simulink model "TxSteering_RxMVDR_4x4_HDL_IQ"  (R2020a)
settings: Solver=FixedStepDiscrete  StartTime=0.0  StopTime=stoptime*0 + inf  RelTol=1e-3
PreLoadFcn:
  | load('iq_bus_obj.mat');
  | model_init
InitFcn:
  | model_init
model workspace (MAT data in the model file):
  socvcb : containers.Map (value not decoded)
values from neighbouring files (symbols this model uses):
  BackSubstitutePrototype = fi(0, matrixdivbacksub_dt)    [model_init.m]
  DataSampleRate = ConverterSampleRate/DecimInterpFactor    (= 245760000)    [model_init.m]
  fc = ConverterSampleRate/4    (= 491520000)    [model_init.m]
  FPGAClkRate = DataSampleRate/VectorSamplingFactor    (= 245760000)    [model_init.m]
  matrixDivDelay = NumberOfCORDICIterations*10 + 86    [model_init.m]
  movavg_bitshift = nextpow2(sqrt(windowSize))    [model_init.m]
  mvdrPipelineDelay = covMatDelay+movAvgDelay+matrixDivDelay+normResponseDelay    [model_init.m]
  NCO_bits = 14    [model_init.m]
  numArrayElements = 4    [model_init.m]
  NumberOfCORDICIterations = matrixdivin_dt.WordLength - 1    [model_init.m]
  S2MM_frame_size = FrameSize*4    (= 40000)    [host_io_init.m]    (also in model_init.m = 1000)
  windowSize = 1024    [model_init.m]
undefined symbols (not defined in the file or in its folder): Fo, Fs, N, physconst
libraries: hdlsllib x268, simulink x53, dspsolvers x1, embreciprocals x1, dsphdlsigops x1
(part 3 of 12)

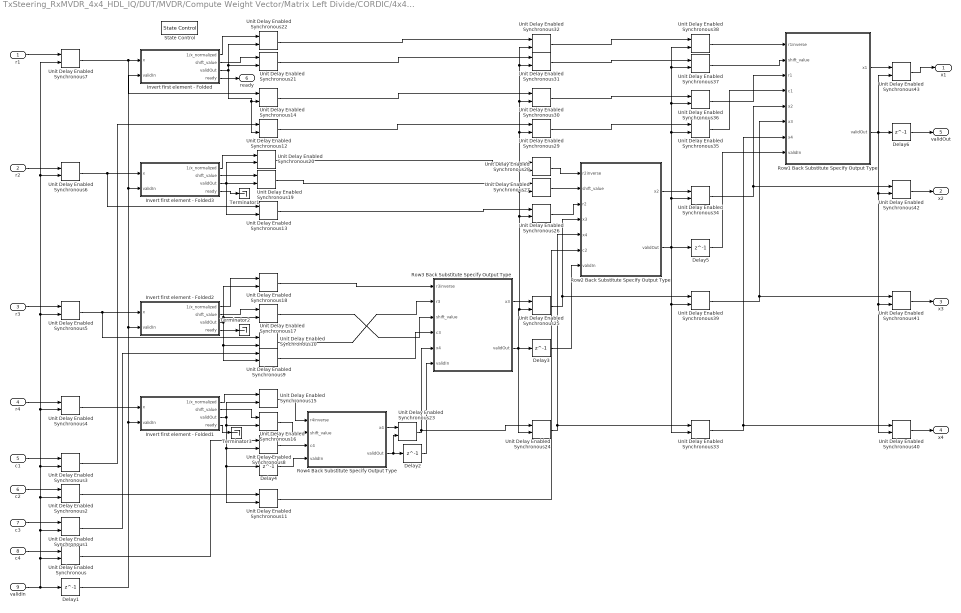
== system TxSteering_RxMVDR_4x4_HDL_IQ/DUT/MVDR/Compute Weight Vector/Matrix Left Divide/CORDIC/4x4 Complex CORDIC Matrix Left Divide/Back Substitute 4x4 Complex CORDIC ==
  r1 : Inport
  r2 : Inport  Port=2
  r3 : Inport  Port=3
  r4 : Inport  Port=4
  c1 : Inport  Port=5
  c2 : Inport  Port=6
  c3 : Inport  Port=7
  c4 : Inport  Port=8
  validIn : Inport  Port=9
  Delay{1..6} (6 alike) : Delay  DelayLength=1
  Invert first element - Folded : Subsystem  TreatAsAtomicUnit=on  mask{NumberOfCORDICIterations=NumberOfCORDICIterations}
      mask prompts: NumberOfCORDICIterations "Number of CORDIC Iterations"
      mask Display: disp('y = 1/x(1)')
  Invert first element - Folded1 : Subsystem  TreatAsAtomicUnit=on  mask{NumberOfCORDICIterations=NumberOfCORDICIterations}
      mask prompts: NumberOfCORDICIterations "Number of CORDIC Iterations"
      mask Display: disp('y = 1/x(1)')
  Invert first element - Folded2 : Subsystem  TreatAsAtomicUnit=on  mask{NumberOfCORDICIterations=NumberOfCORDICIterations}
      mask prompts: NumberOfCORDICIterations "Number of CORDIC Iterations"
      mask Display: disp('y = 1/x(1)')
  Invert first element - Folded3 : Subsystem  TreatAsAtomicUnit=on  mask{NumberOfCORDICIterations=NumberOfCORDICIterations}
      mask prompts: NumberOfCORDICIterations "Number of CORDIC Iterations"
      mask Display: disp('y = 1/x(1)')
  Row1 Back Substitute Specify Output Type : Subsystem  TreatAsAtomicUnit=on
  Row2 Back Substitute Specify Output Type : Subsystem  TreatAsAtomicUnit=on
  Row3 Back Substitute Specify Output Type : Subsystem  TreatAsAtomicUnit=on
  Row4 Back Substitute Specify Output Type : Subsystem  TreatAsAtomicUnit=on
  State Control : StateControl  StateControl=Synchronous
  Terminator1 : Terminator
  Terminator2 : Terminator
  Terminator3 : Terminator
  Unit Delay Enabled Synchronous{,1..43} (44 alike) : hdlsllib/Discrete/Unit Delay Enabled Synchronous  InitialCondition=0.0  SampleTime=-1
      settings: SourceProductBaseCode=SL
  x1 : Outport  VectorParamsAs1DForOutWhenUnconnected=off
  x2 : Outport  Port=2  VectorParamsAs1DForOutWhenUnconnected=off
  x3 : Outport  Port=3  VectorParamsAs1DForOutWhenUnconnected=off
  x4 : Outport  Port=4  VectorParamsAs1DForOutWhenUnconnected=off
  validOut : Outport  Port=5  VectorParamsAs1DForOutWhenUnconnected=off
  ready : Outport  Port=6  VectorParamsAs1DForOutWhenUnconnected=off
  wires:
  Invert first element - Folded/1(1/x_normalized) -> Unit Delay Enabled Synchronous22/1
  Invert first element - Folded1/1(1/x_normalized) -> Unit Delay Enabled Synchronous15/1
  Unit Delay Enabled Synchronous40/1 -> x4/1
  Unit Delay Enabled Synchronous41/1 -> x3/1
  Unit Delay Enabled Synchronous42/1 -> x2/1
  Unit Delay Enabled Synchronous43/1 -> x1/1
  Invert first element - Folded/2(shift_value) -> Unit Delay Enabled Synchronous21/1
  validIn/1 -> Unit Delay Enabled Synchronous/2, Unit Delay Enabled Synchronous1/2, Unit Delay Enabled Synchronous2/2, Unit Delay Enabled Synchronous3/2, Unit Delay Enabled Synchronous4/2, Unit Delay Enabled Synchronous6/2, Unit Delay Enabled Synchronous7/2, Unit Delay Enabled Synchronous5/2, Delay1/1
  Invert first element - Folded3/1(1/x_normalized) -> Unit Delay Enabled Synchronous20/1
  Invert first element - Folded2/1(1/x_normalized) -> Unit Delay Enabled Synchronous18/1
  Invert first element - Folded2/2(shift_value) -> Unit Delay Enabled Synchronous17/1
  Invert first element - Folded3/2(shift_value) -> Unit Delay Enabled Synchronous19/1
  Invert first element - Folded1/2(shift_value) -> Unit Delay Enabled Synchronous16/1
  Unit Delay Enabled Synchronous7/1 -> Unit Delay Enabled Synchronous14/1, Invert first element - Folded/1(x)
  Unit Delay Enabled Synchronous6/1 -> Unit Delay Enabled Synchronous13/1, Invert first element - Folded3/1(x)
  Unit Delay Enabled Synchronous5/1 -> Unit Delay Enabled Synchronous10/1, Invert first element - Folded2/1(x)
  Unit Delay Enabled Synchronous4/1 -> Invert first element - Folded1/1(x)
  Unit Delay Enabled Synchronous3/1 -> Unit Delay Enabled Synchronous12/1
  Unit Delay Enabled Synchronous2/1 -> Unit Delay Enabled Synchronous11/1
  Unit Delay Enabled Synchronous1/1 -> Unit Delay Enabled Synchronous9/1
  Delay1/1 -> Invert first element - Folded1/2(validIn), Invert first element - Folded/2(validIn), Invert first element - Folded3/2(validIn), Invert first element - Folded2/2(validIn)
  Unit Delay Enabled Synchronous28/1 -> Row2 Back Substitute Specify Output Type/1(r2inverse)
  Unit Delay Enabled Synchronous27/1 -> Row2 Back Substitute Specify Output Type/2(shift_value)
  Unit Delay Enabled Synchronous26/1 -> Row2 Back Substitute Specify Output Type/3(r2)
  Unit Delay Enabled Synchronous11/1 -> Row2 Back Substitute Specify Output Type/6(c2)
  Row2 Back Substitute Specify Output Type/1(x2) -> Unit Delay Enabled Synchronous34/1
  Unit Delay Enabled Synchronous18/1 -> Row3 Back Substitute Specify Output Type/1(r3inverse)
  Unit Delay Enabled Synchronous10/1 -> Row3 Back Substitute Specify Output Type/2(r3)
  Unit Delay Enabled Synchronous17/1 -> Row3 Back Substitute Specify Output Type/3(shift_value)
  Unit Delay Enabled Synchronous9/1 -> Row3 Back Substitute Specify Output Type/4(c3)
  Row3 Back Substitute Specify Output Type/1(x3) -> Unit Delay Enabled Synchronous25/1
  Unit Delay Enabled Synchronous15/1 -> Row4 Back Substitute Specify Output Type/1(r4inverse)
  Unit Delay Enabled Synchronous16/1 -> Row4 Back Substitute Specify Output Type/2(shift_value)
  Unit Delay Enabled Synchronous8/1 -> Row4 Back Substitute Specify Output Type/3(c4)
  Unit Delay Enabled Synchronous38/1 -> Row1 Back Substitute Specify Output Type/1(r1inverse)
  Unit Delay Enabled Synchronous37/1 -> Row1 Back Substitute Specify Output Type/2(shift_value)
  Unit Delay Enabled Synchronous36/1 -> Row1 Back Substitute Specify Output Type/3(r1)
  Unit Delay Enabled Synchronous35/1 -> Row1 Back Substitute Specify Output Type/4(c1)
  Row1 Back Substitute Specify Output Type/1(x1) -> Unit Delay Enabled Synchronous43/1
  Unit Delay Enabled Synchronous23/1 -> Unit Delay Enabled Synchronous24/1, Row3 Back Substitute Specify Output Type/5(x4)
  Unit Delay Enabled Synchronous13/1 -> Unit Delay Enabled Synchronous26/1
  Unit Delay Enabled Synchronous20/1 -> Unit Delay Enabled Synchronous28/1
  Unit Delay Enabled Synchronous12/1 -> Unit Delay Enabled Synchronous29/1
  Unit Delay Enabled Synchronous14/1 -> Unit Delay Enabled Synchronous30/1
  Unit Delay Enabled Synchronous21/1 -> Unit Delay Enabled Synchronous31/1
  Unit Delay Enabled Synchronous22/1 -> Unit Delay Enabled Synchronous32/1
  Unit Delay Enabled Synchronous25/1 -> Unit Delay Enabled Synchronous39/1, Row2 Back Substitute Specify Output Type/4(x3)
  Unit Delay Enabled Synchronous24/1 -> Unit Delay Enabled Synchronous33/1, Row2 Back Substitute Specify Output Type/5(x4)
  Unit Delay Enabled Synchronous29/1 -> Unit Delay Enabled Synchronous35/1
  Unit Delay Enabled Synchronous30/1 -> Unit Delay Enabled Synchronous36/1
  Unit Delay Enabled Synchronous31/1 -> Unit Delay Enabled Synchronous37/1
  Unit Delay Enabled Synchronous32/1 -> Unit Delay Enabled Synchronous38/1
  Unit Delay Enabled Synchronous34/1 -> Row1 Back Substitute Specify Output Type/5(x2), Unit Delay Enabled Synchronous42/1
  Unit Delay Enabled Synchronous39/1 -> Unit Delay Enabled Synchronous41/1, Row1 Back Substitute Specify Output Type/6(x3)
  Unit Delay Enabled Synchronous33/1 -> Unit Delay Enabled Synchronous40/1, Row1 Back Substitute Specify Output Type/7(x4)
  Invert first element - Folded/4(ready) -> ready/1
  Invert first element - Folded/3(validOut) -> Unit Delay Enabled Synchronous21/2, Unit Delay Enabled Synchronous22/2, Unit Delay Enabled Synchronous14/2, Unit Delay Enabled Synchronous12/2
  Invert first element - Folded1/4(ready) -> Terminator3/1
  Invert first element - Folded2/4(ready) -> Terminator2/1
  Invert first element - Folded3/4(ready) -> Terminator1/1
  Invert first element - Folded3/3(validOut) -> Unit Delay Enabled Synchronous19/2, Unit Delay Enabled Synchronous20/2, Unit Delay Enabled Synchronous13/2
  c4/1 -> Unit Delay Enabled Synchronous/1
  c3/1 -> Unit Delay Enabled Synchronous1/1
  c2/1 -> Unit Delay Enabled Synchronous2/1
  c1/1 -> Unit Delay Enabled Synchronous3/1
  r4/1 -> Unit Delay Enabled Synchronous4/1
  r3/1 -> Unit Delay Enabled Synchronous5/1
  r2/1 -> Unit Delay Enabled Synchronous6/1
  r1/1 -> Unit Delay Enabled Synchronous7/1
  Row4 Back Substitute Specify Output Type/2(validOut) -> Unit Delay Enabled Synchronous23/2, Delay2/1
  Delay4/1 -> Row4 Back Substitute Specify Output Type/4(validIn)
  Unit Delay Enabled Synchronous/1 -> Unit Delay Enabled Synchronous8/1
  Row4 Back Substitute Specify Output Type/1(x4) -> Unit Delay Enabled Synchronous23/1
  Invert first element - Folded2/3(validOut) -> Unit Delay Enabled Synchronous18/2, Unit Delay Enabled Synchronous17/2, Unit Delay Enabled Synchronous10/2, Unit Delay Enabled Synchronous9/2
  Invert first element - Folded1/3(validOut) -> Unit Delay Enabled Synchronous16/2, Unit Delay Enabled Synchronous11/2, Delay4/1, Unit Delay Enabled Synchronous8/2, Unit Delay Enabled Synchronous15/2
  Row3 Back Substitute Specify Output Type/2(validOut) -> Unit Delay Enabled Synchronous26/2, Unit Delay Enabled Synchronous27/2, Unit Delay Enabled Synchronous28/2, Unit Delay Enabled Synchronous29/2, Unit Delay Enabled Synchronous30/2, Unit Delay Enabled Synchronous31/2, Unit Delay Enabled Synchronous32/2, Unit Delay Enabled Synchronous25/2, Unit Delay Enabled Synchronous24/2, Delay3/1
  Row2 Back Substitute Specify Output Type/2(validOut) -> Unit Delay Enabled Synchronous33/2, Unit Delay Enabled Synchronous39/2, Unit Delay Enabled Synchronous34/2, Unit Delay Enabled Synchronous35/2, Unit Delay Enabled Synchronous36/2, Unit Delay Enabled Synchronous38/2, Unit Delay Enabled Synchronous37/2, Delay5/1
  Delay2/1 -> Row3 Back Substitute Specify Output Type/6(validIn)
  Delay3/1 -> Row2 Back Substitute Specify Output Type/7(validIn)
  Delay5/1 -> Row1 Back Substitute Specify Output Type/8(validIn)
  Delay6/1 -> validOut/1
  Unit Delay Enabled Synchronous19/1 -> Unit Delay Enabled Synchronous27/1
  Row1 Back Substitute Specify Output Type/2(validOut) -> Unit Delay Enabled Synchronous42/2, Unit Delay Enabled Synchronous41/2, Unit Delay Enabled Synchronous40/2, Unit Delay Enabled Synchronous43/2, Delay6/1

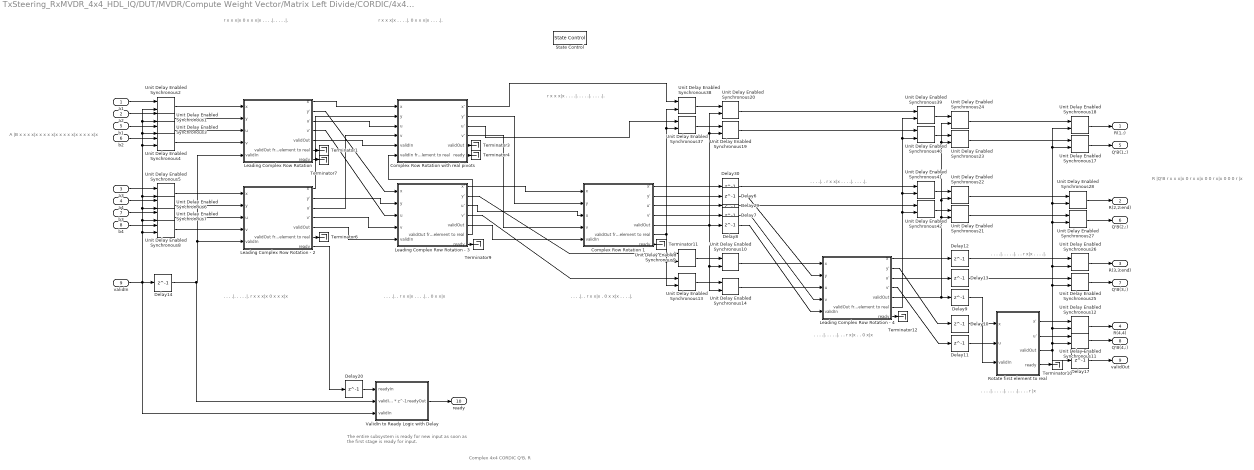
== system TxSteering_RxMVDR_4x4_HDL_IQ/DUT/MVDR/Compute Weight Vector/Matrix Left Divide/CORDIC/4x4 Complex CORDIC Matrix Left Divide/Q'B, R 4x4 Complex CORDIC Systolic Array ==
  note: The entire subsystem is ready for new input as soon
      | as the first stage is ready for input.
  note: . . . .|.
      | . . . .|.
      | . . r x|x
      | . . . .|.
  note: . . . .|.
      | . r x x|x
      | . . . .|.
      | . . . .|.
  note: R |Q'B
      | r x x x|x
      | 0 r x x|x
      | 0 0 r x|x
      | 0 0 0 r |x
  note: r x x x|x
      | . . . .|.
      | . . . .|.
      | . . . .|.
  note: . . . .|.
      | . . . .|.
      | . . . .|.
      | . . . r |x
  note: . . . .|.
      | . . . .|.
      | . . r x|x
      | . . 0 x|x
  note: . . . .|.
      | . r x x|x
      | . . . .|.
      | . 0 x x|x
  note: . . . .|.
      | . r x x|x
      | . 0 x x|x
      | . . . .|.
  note: . . . .|.
      | . . . .|.
      | r x x x|x
      | 0 x x x|x
  note: r x x x|x
      | . . . .|.
      | 0 x x x|x
      | . . . .|.
  note: A |B
      | x x x x|x
      | x x x x|x
      | x x x x|x
      | x x x x|x
  note: Complex 4x4 CORDIC Q'B, R
  note: r x x x|x
      | 0 x x x|x
      | . . . .|.
      | . . . .|.
  a1 : Inport
  a2 : Inport  Port=2
  a3 : Inport  Port=3
  a4 : Inport  Port=4
  b1 : Inport  Port=5
  b2 : Inport  Port=6
  b3 : Inport  Port=7
  b4 : Inport  Port=8
  validIn : Inport  Port=9
  Complex Row Rotation with real pivots : Subsystem  TreatAsAtomicUnit=on  mask{NumberOfCORDICIterations=NumberOfCORDICIterations}
      mask prompts: NumberOfCORDICIterations "Number of CORDIC Iterations"
  Complex Row Rotation 1 : Subsystem  TreatAsAtomicUnit=on  mask{NumberOfCORDICIterations=NumberOfCORDICIterations}
      mask prompts: NumberOfCORDICIterations "Number of CORDIC Iterations"
  Delay{6..14,17,29..30} (12 alike) : Delay  DelayLength=1
  Delay20 : Delay  DelayLength=1  InitialCondition=true
  Leading Complex Row Rotation : Subsystem  TreatAsAtomicUnit=on  mask{NumberOfCORDICIterations=NumberOfCORDICIterations}
      mask prompts: NumberOfCORDICIterations "Number of CORDIC Iterations"
  Leading Complex Row Rotation - 2 : Subsystem  TreatAsAtomicUnit=on  mask{NumberOfCORDICIterations=NumberOfCORDICIterations}
      mask prompts: NumberOfCORDICIterations "Number of CORDIC Iterations"
  Leading Complex Row Rotation - 3 : Subsystem  TreatAsAtomicUnit=on  mask{NumberOfCORDICIterations=NumberOfCORDICIterations}
      mask prompts: NumberOfCORDICIterations "Number of CORDIC Iterations"
  Leading Complex Row Rotation - 4 : Subsystem  TreatAsAtomicUnit=on  mask{NumberOfCORDICIterations=NumberOfCORDICIterations}
      mask prompts: NumberOfCORDICIterations "Number of CORDIC Iterations"
  Rotate first element to real : Subsystem  TreatAsAtomicUnit=on  mask{NumberOfCORDICIterations=NumberOfCORDICIterations}
      mask prompts: NumberOfCORDICIterations "Number of CORDIC Iterations"
  State Control : StateControl  StateControl=Synchronous
  Terminator{1,3..4,6..7,9..12} (9 alike) : Terminator
  Unit Delay Enabled Synchronous{1..14,17..28,37..42} (32 alike) : hdlsllib/Discrete/Unit Delay Enabled Synchronous  InitialCondition=0.0  SampleTime=-1
      settings: SourceProductBaseCode=SL
  ValidIn to Ready Logic with Delay : Subsystem
  R(1,:) : Outport  VectorParamsAs1DForOutWhenUnconnected=off
  R(2,2:end) : Outport  Port=2  VectorParamsAs1DForOutWhenUnconnected=off
  R(3,3:end) : Outport  Port=3  VectorParamsAs1DForOutWhenUnconnected=off
  R(4,4) : Outport  Port=4  VectorParamsAs1DForOutWhenUnconnected=off
  Q'B(1,:) : Outport  Port=5  VectorParamsAs1DForOutWhenUnconnected=off
  Q'B(2,:) : Outport  Port=6  VectorParamsAs1DForOutWhenUnconnected=off
  Q'B(3,:) : Outport  Port=7  VectorParamsAs1DForOutWhenUnconnected=off
  Q'B(4,:) : Outport  Port=8  VectorParamsAs1DForOutWhenUnconnected=off
  validOut : Outport  Port=9  VectorParamsAs1DForOutWhenUnconnected=off
  ready : Outport  Port=10  VectorParamsAs1DForOutWhenUnconnected=off
  wires:
  Leading Complex Row Rotation - 4/4(v') -> Delay11/1
  Unit Delay Enabled Synchronous40/1 -> Unit Delay Enabled Synchronous23/1
  Leading Complex Row Rotation - 4/6(validOut from rotate first element to real) -> Unit Delay Enabled Synchronous42/2, Unit Delay Enabled Synchronous40/2, Unit Delay Enabled Synchronous39/2, Unit Delay Enabled Synchronous41/2
  Complex Row Rotation 1/2(y') -> Delay6/1
  Unit Delay Enabled Synchronous37/1 -> Unit Delay Enabled Synchronous19/1
  Leading Complex Row Rotation - 3/1(x') -> Complex Row Rotation 1/1(x)
  Leading Complex Row Rotation - 3/4(v') -> Unit Delay Enabled Synchronous13/1
  Complex Row Rotation with real pivots/4(v') -> Complex Row Rotation 1/4(v)
  Complex Row Rotation with real pivots/1(x') -> Unit Delay Enabled Synchronous38/1
  Leading Complex Row Rotation - 2/5(validOut) -> Leading Complex Row Rotation - 3/5(validIn)
  Leading Complex Row Rotation - 2/4(v') -> Leading Complex Row Rotation - 3/4(v)
  Leading Complex Row Rotation/5(validOut) -> Complex Row Rotation with real pivots/5(validIn)
  Leading Complex Row Rotation/2(y') -> Leading Complex Row Rotation - 3/1(x)
  Leading Complex Row Rotation/3(u') -> Complex Row Rotation with real pivots/3(u)
  Delay20/1 -> ValidIn to Ready Logic with Delay/1(readyIn)
  Leading Complex Row Rotation - 3/2(y') -> Unit Delay Enabled Synchronous9/1
  Unit Delay Enabled Synchronous14/1 -> Leading Complex Row Rotation - 4/3(u)
  Unit Delay Enabled Synchronous13/1 -> Unit Delay Enabled Synchronous14/1
  Unit Delay Enabled Synchronous10/1 -> Leading Complex Row Rotation - 4/1(x)
  Unit Delay Enabled Synchronous9/1 -> Unit Delay Enabled Synchronous10/1
  Leading Complex Row Rotation - 2/7(ready) -> Delay20/1
  Leading Complex Row Rotation/4(v') -> Leading Complex Row Rotation - 3/3(u)
  Leading Complex Row Rotation - 2/2(y') -> Leading Complex Row Rotation - 3/2(y)
  Leading Complex Row Rotation - 2/3(u') -> Complex Row Rotation with real pivots/4(v)
  Leading Complex Row Rotation - 2/1(x') -> Complex Row Rotation with real pivots/2(y)
  Leading Complex Row Rotation/1(x') -> Complex Row Rotation with real pivots/1(x)
  Complex Row Rotation with real pivots/3(u') -> Unit Delay Enabled Synchronous37/1
  Complex Row Rotation with real pivots/6(ready) -> Terminator4/1
  Complex Row Rotation with real pivots/5(validOut) -> Terminator3/1
  Unit Delay Enabled Synchronous18/1 -> R(1,:)/1
  Leading Complex Row Rotation - 3/6(validOut from rotate first element to real) -> Complex Row Rotation with real pivots/6(validIn from rotate first element to real)
  Delay11/1 -> Rotate first element to real/2(u)
  Delay10/1 -> Rotate first element to real/1(x)
  Leading Complex Row Rotation - 4/2(y') -> Delay10/1
  Unit Delay Enabled Synchronous42/1 -> Unit Delay Enabled Synchronous21/1
  Delay29/1 -> Unit Delay Enabled Synchronous42/1
  Unit Delay Enabled Synchronous41/1 -> Unit Delay Enabled Synchronous22/1
  Delay30/1 -> Unit Delay Enabled Synchronous41/1
  Unit Delay Enabled Synchronous19/1 -> Unit Delay Enabled Synchronous40/1
  Unit Delay Enabled Synchronous39/1 -> Unit Delay Enabled Synchronous24/1
  Unit Delay Enabled Synchronous20/1 -> Unit Delay Enabled Synchronous39/1
  Delay9/1 -> Rotate first element to real/3(validIn)
  Complex Row Rotation 1/6(validOut from rotate first element to real) -> Unit Delay Enabled Synchronous38/2, Unit Delay Enabled Synchronous37/2, Unit Delay Enabled Synchronous9/2, Unit Delay Enabled Synchronous13/2
  Unit Delay Enabled Synchronous38/1 -> Unit Delay Enabled Synchronous20/1
  Complex Row Rotation 1/3(u') -> Delay29/1
  Complex Row Rotation 1/1(x') -> Delay30/1
  Delay8/1 -> Leading Complex Row Rotation - 4/5(validIn)
  Delay7/1 -> Leading Complex Row Rotation - 4/4(v)
  Complex Row Rotation 1/4(v') -> Delay7/1
  Delay6/1 -> Leading Complex Row Rotation - 4/2(y)
  Complex Row Rotation with real pivots/2(y') -> Complex Row Rotation 1/2(y)
  Leading Complex Row Rotation - 3/5(validOut) -> Complex Row Rotation 1/5(validIn)
  Leading Complex Row Rotation - 3/3(u') -> Complex Row Rotation 1/3(u)
  Leading Complex Row Rotation - 4/7(ready) -> Terminator12/1
  Complex Row Rotation 1/7(ready) -> Terminator11/1
  Leading Complex Row Rotation - 3/7(ready) -> Terminator9/1
  Leading Complex Row Rotation/6(validOut from rotate first element to real) -> Terminator1/1
  Leading Complex Row Rotation/7(ready) -> Terminator7/1
  Leading Complex Row Rotation - 2/6(validOut from rotate first element to real) -> Terminator6/1
  Unit Delay Enabled Synchronous25/1 -> Q'B(3,:)/1
  Delay13/1 -> Unit Delay Enabled Synchronous25/1
  Unit Delay Enabled Synchronous26/1 -> R(3,3:end)/1
  Delay12/1 -> Unit Delay Enabled Synchronous26/1
  Unit Delay Enabled Synchronous27/1 -> Q'B(2,:)/1
  Unit Delay Enabled Synchronous21/1 -> Unit Delay Enabled Synchronous27/1
  Unit Delay Enabled Synchronous28/1 -> R(2,2:end)/1
  Unit Delay Enabled Synchronous22/1 -> Unit Delay Enabled Synchronous28/1
  Unit Delay Enabled Synchronous23/1 -> Unit Delay Enabled Synchronous17/1
  Unit Delay Enabled Synchronous24/1 -> Unit Delay Enabled Synchronous18/1
  ValidIn to Ready Logic with Delay/1(readyOut) -> ready/1
  b4/1 -> Unit Delay Enabled Synchronous8/1
  b3/1 -> Unit Delay Enabled Synchronous7/1
  a4/1 -> Unit Delay Enabled Synchronous6/1
  a3/1 -> Unit Delay Enabled Synchronous5/1
  b2/1 -> Unit Delay Enabled Synchronous4/1
  b1/1 -> Unit Delay Enabled Synchronous3/1
  a2/1 -> Unit Delay Enabled Synchronous1/1
  a1/1 -> Unit Delay Enabled Synchronous2/1
  validIn/1 -> Delay14/1, Unit Delay Enabled Synchronous2/2, Unit Delay Enabled Synchronous1/2, Unit Delay Enabled Synchronous3/2, Unit Delay Enabled Synchronous4/2, Unit Delay Enabled Synchronous5/2, Unit Delay Enabled Synchronous6/2, Unit Delay Enabled Synchronous7/2, Unit Delay Enabled Synchronous8/2, ValidIn to Ready Logic with Delay/3(validIn)
  Unit Delay Enabled Synchronous17/1 -> Q'B(1,:)/1
  Leading Complex Row Rotation - 4/3(u') -> Delay13/1
  Leading Complex Row Rotation - 4/1(x') -> Delay12/1
  Complex Row Rotation 1/5(validOut) -> Delay8/1, Unit Delay Enabled Synchronous14/2, Unit Delay Enabled Synchronous10/2, Unit Delay Enabled Synchronous19/2, Unit Delay Enabled Synchronous20/2
  Leading Complex Row Rotation - 4/5(validOut) -> Unit Delay Enabled Synchronous21/2, Unit Delay Enabled Synchronous24/2, Unit Delay Enabled Synchronous23/2, Unit Delay Enabled Synchronous22/2, Delay9/1
  Delay14/1 -> Leading Complex Row Rotation/5(validIn), Leading Complex Row Rotation - 2/5(validIn), ValidIn to Ready Logic with Delay/2(validIn * z^-1)
  Unit Delay Enabled Synchronous8/1 -> Leading Complex Row Rotation - 2/4(v)
  Unit Delay Enabled Synchronous7/1 -> Leading Complex Row Rotation - 2/3(u)
  Unit Delay Enabled Synchronous6/1 -> Leading Complex Row Rotation - 2/2(y)
  Unit Delay Enabled Synchronous5/1 -> Leading Complex Row Rotation - 2/1(x)
  Unit Delay Enabled Synchronous4/1 -> Leading Complex Row Rotation/4(v)
  Unit Delay Enabled Synchronous3/1 -> Leading Complex Row Rotation/3(u)
  Unit Delay Enabled Synchronous1/1 -> Leading Complex Row Rotation/2(y)
  Unit Delay Enabled Synchronous2/1 -> Leading Complex Row Rotation/1(x)
  Rotate first element to real/4(ready) -> Terminator10/1
  Unit Delay Enabled Synchronous12/1 -> R(4,4)/1
  Unit Delay Enabled Synchronous11/1 -> Q'B(4,:)/1
  Delay17/1 -> validOut/1
  Rotate first element to real/3(validOut) -> Delay17/1, Unit Delay Enabled Synchronous27/2, Unit Delay Enabled Synchronous28/2, Unit Delay Enabled Synchronous18/2, Unit Delay Enabled Synchronous17/2, Unit Delay Enabled Synchronous26/2, Unit Delay Enabled Synchronous25/2, Unit Delay Enabled Synchronous12/2, Unit Delay Enabled Synchronous11/2
  Rotate first element to real/2(u') -> Unit Delay Enabled Synchronous11/1
  Rotate first element to real/1(x') -> Unit Delay Enabled Synchronous12/1

== system TxSteering_RxMVDR_4x4_HDL_IQ/DUT/MVDR/Compute Weight Vector/Matrix Left Divide/CORDIC/4x4 Complex CORDIC Matrix Left Divide/ValidIn to Ready Logic with Delay ==
  readyIn : Inport
  validIn * z^-1 : Inport  Port=2
  validIn : Inport  Port=3
  AND : Logic  IconShape=distinctive  AllPortsSameDT=off  OutDataTypeStr=boolean
  AND1 : Logic  IconShape=distinctive  AllPortsSameDT=off  OutDataTypeStr=boolean
  NOT : Logic  Operator=NOT  IconShape=distinctive  AllPortsSameDT=off  OutDataTypeStr=boolean
  NOT1 : Logic  Operator=NOT  IconShape=distinctive  AllPortsSameDT=off  OutDataTypeStr=boolean
  readyOut : Outport  VectorParamsAs1DForOutWhenUnconnected=off
  wires:
  validIn * z^-1/1 -> NOT/1
  validIn/1 -> NOT1/1
  readyIn/1 -> AND/1
  AND1/1 -> readyOut/1
  NOT1/1 -> AND1/2
  NOT/1 -> AND/2
  AND/1 -> AND1/1

== system TxSteering_RxMVDR_4x4_HDL_IQ/DUT/MVDR/Form Covariance Matrix/Matrix Multiply Partitioned/Partition x_conj/Partition x/HDL Complex Multiply ==
  note: Xilinx devices:
      | - Set D1 = 1 or 2 to trade off speed & FF resources
      | - Set D2-D5 = 1 to fully leverage DSP48 pipelines
      | - Use sync reset
      |
      | Intel FPGAs:
      | - Set D1 = 1 or 2 depending on device family
      | - Set D5 = 1; D2, D3, D4 = 0
      | - Use async reset
  In1 : Inport
  In2 : Inport  Port=2
  Add1 : Sum
  Add2 : Sum  Inputs=+-
  Add3 : Sum
  Add4 : Sum  Inputs=-+
  Add5 : Sum
  Complex to Real-Imag : ComplexToRealImag
  Complex to Real-Imag1 : ComplexToRealImag
  D1_1 : Delay  DelayLength=D1
  D1_2 : Delay  DelayLength=D1
  D2_{1..6} (6 alike) : Delay  DelayLength=D2
  D3_{1..5} (5 alike) : Delay  DelayLength=D3
  D4_1 : Delay  DelayLength=D4
  D4_2 : Delay  DelayLength=D4
  D4_3 : Delay  DelayLength=D4
  D5_1 : Delay  DelayLength=D5
  D5_2 : Delay  DelayLength=D5
  Product1 : Product
  Product2 : Product
  Product3 : Product
  Real-Imag to Complex : RealImagToComplex
  Out1 : Outport  VectorParamsAs1DForOutWhenUnconnected=off
  wires:
  Real-Imag to Complex/1 -> Out1/1
  In2/1 -> D1_2/1
  Complex to Real-Imag1/1 -> Add3/1, D2_4/1  "C"
  Complex to Real-Imag1/2 -> Add3/2, D2_3/1  "D"
  Product1/1 -> D4_1/1  "X"
  Product2/1 -> D4_2/1  "Y"
  Product3/1 -> D3_5/1  "Z"
  Add4/1 -> D5_1/1
  Add5/1 -> D5_2/1
  D5_1/1 -> Real-Imag to Complex/1
  D5_2/1 -> Real-Imag to Complex/2
  D4_1/1 -> Add4/1
  D4_2/1 -> Add5/1
  D3_5/1 -> D4_3/1
  Add1/1 -> D3_1/1
  Add3/1 -> D2_6/1
  Add2/1 -> D3_3/1
  Complex to Real-Imag/1 -> D2_5/1, D2_1/1  "A"
  Complex to Real-Imag/2 -> D2_2/1  "B"
  D3_1/1 -> Product1/1
  D2_6/1 -> Product3/2
  D3_3/1 -> Product2/1
  D4_3/1 -> Add4/2, Add5/2
  D3_4/1 -> Product2/2
  D3_2/1 -> Product1/2
  D2_4/1 -> D3_4/1
  D2_3/1 -> D3_2/1
  D2_5/1 -> Product3/1
  D2_2/1 -> Add1/2, Add2/1
  D2_1/1 -> Add2/2, Add1/1
  In1/1 -> D1_1/1
  D1_1/1 -> Complex to Real-Imag/1
  D1_2/1 -> Complex to Real-Imag1/1

== system TxSteering_RxMVDR_4x4_HDL_IQ/DUT/MVDR/Normalize Response/MVDR Weight Update/Inner Product/Element-wise complex product/HDL Complex Multiply ==
  note: Xilinx devices:
      | - Set D1 = 1 or 2 to trade off speed & FF resources
      | - Set D2-D5 = 1 to fully leverage DSP48 pipelines
      | - Use sync reset
      |
      | Intel FPGAs:
      | - Set D1 = 1 or 2 depending on device family
      | - Set D5 = 1; D2, D3, D4 = 0
      | - Use async reset
  In1 : Inport
  In2 : Inport  Port=2
  Add1 : Sum
  Add2 : Sum  Inputs=+-
  Add3 : Sum
  Add4 : Sum  Inputs=-+
  Add5 : Sum
  Complex to Real-Imag : ComplexToRealImag
  Complex to Real-Imag1 : ComplexToRealImag
  D1_1 : Delay  DelayLength=D1
  D1_2 : Delay  DelayLength=D1
  D2_{1..6} (6 alike) : Delay  DelayLength=D2
  D3_{1..5} (5 alike) : Delay  DelayLength=D3
  D4_1 : Delay  DelayLength=D4
  D4_2 : Delay  DelayLength=D4
  D4_3 : Delay  DelayLength=D4
  D5_1 : Delay  DelayLength=D5
  D5_2 : Delay  DelayLength=D5
  Product1 : Product  OutDataTypeStr=Inherit: Same as first input
  Product2 : Product  OutDataTypeStr=Inherit: Same as first input
  Product3 : Product  OutDataTypeStr=Inherit: Same as first input
  Real-Imag to Complex : RealImagToComplex
  Out1 : Outport  VectorParamsAs1DForOutWhenUnconnected=off
  wires:
  Real-Imag to Complex/1 -> Out1/1
  In2/1 -> D1_2/1
  Complex to Real-Imag1/1 -> Add3/1, D2_4/1  "C"
  Complex to Real-Imag1/2 -> Add3/2, D2_3/1  "D"
  Product1/1 -> D4_1/1  "X"
  Product2/1 -> D4_2/1  "Y"
  Product3/1 -> D3_5/1  "Z"
  Add4/1 -> D5_1/1
  Add5/1 -> D5_2/1
  D5_1/1 -> Real-Imag to Complex/1
  D5_2/1 -> Real-Imag to Complex/2
  D4_1/1 -> Add4/1
  D4_2/1 -> Add5/1
  D3_5/1 -> D4_3/1
  Add1/1 -> D3_1/1
  Add3/1 -> D2_6/1
  Add2/1 -> D3_3/1
  Complex to Real-Imag/1 -> D2_5/1, D2_1/1  "A"
  Complex to Real-Imag/2 -> D2_2/1  "B"
  D3_1/1 -> Product1/1
  D2_6/1 -> Product3/2
  D3_3/1 -> Product2/1
  D4_3/1 -> Add4/2, Add5/2
  D3_4/1 -> Product2/2
  D3_2/1 -> Product1/2
  D2_4/1 -> D3_4/1
  D2_3/1 -> D3_2/1
  D2_5/1 -> Product3/1
  D2_2/1 -> Add1/2, Add2/1
  D2_1/1 -> Add2/2, Add1/1
  In1/1 -> D1_1/1
  D1_1/1 -> Complex to Real-Imag/1
  D1_2/1 -> Complex to Real-Imag1/1

== system TxSteering_RxMVDR_4x4_HDL_IQ/DUT/MVDR/Compute Weight Vector/Matrix Left Divide/CORDIC/4x4 Complex CORDIC Matrix Left Divide/Back Substitute 4x4 Complex CORDIC/Invert first element - Folded ==
  x : Inport
  validIn : Inport  Port=2
  "CORDIC Reciprocal Normalized, Folded" : Subsystem  TreatAsAtomicUnit=on  mask{NumberOfCORDICIterations=NumberOfCORDICIterations}
      mask prompts: NumberOfCORDICIterations "Number of CORDIC Iterations"
  State Control : StateControl  StateControl=Synchronous
  ValidIn to Ready Logic : Subsystem
  y = x(n) : MATLAB Function  TreatAsAtomicUnit=on  mask{n=1}
  1/x_normalized : Outport  VectorParamsAs1DForOutWhenUnconnected=off
  shift_value : Outport  Port=2  VectorParamsAs1DForOutWhenUnconnected=off
  validOut : Outport  Port=3  VectorParamsAs1DForOutWhenUnconnected=off
  ready : Outport  Port=4  VectorParamsAs1DForOutWhenUnconnected=off
  wires:
  y = x(n)/1(y) -> "CORDIC Reciprocal Normalized, Folded"/1(x)
  "CORDIC Reciprocal Normalized, Folded"/1(1/x_normalized) -> 1/x_normalized/1
  x/1 -> y = x(n)/1(x)
  validIn/1 -> ValidIn to Ready Logic/2(validIn), "CORDIC Reciprocal Normalized, Folded"/2(validIn)
  "CORDIC Reciprocal Normalized, Folded"/3(validOut) -> validOut/1
  "CORDIC Reciprocal Normalized, Folded"/2(shift_value) -> shift_value/1
  "CORDIC Reciprocal Normalized, Folded"/4(ready) -> ValidIn to Ready Logic/1(readyIn)
  ValidIn to Ready Logic/1(readyOut) -> ready/1

== system TxSteering_RxMVDR_4x4_HDL_IQ/DUT/MVDR/Compute Weight Vector/Matrix Left Divide/CORDIC/4x4 Complex CORDIC Matrix Left Divide/Back Substitute 4x4 Complex CORDIC/Invert first element - Folded1 ==
  x : Inport
  validIn : Inport  Port=2
  "CORDIC Reciprocal Normalized, Folded" : Subsystem  TreatAsAtomicUnit=on  mask{NumberOfCORDICIterations=NumberOfCORDICIterations}
      mask prompts: NumberOfCORDICIterations "Number of CORDIC Iterations"
  State Control : StateControl  StateControl=Synchronous
  ValidIn to Ready Logic : Subsystem
  y = x(n) : MATLAB Function  TreatAsAtomicUnit=on  mask{n=1}
  1/x_normalized : Outport  VectorParamsAs1DForOutWhenUnconnected=off
  shift_value : Outport  Port=2  VectorParamsAs1DForOutWhenUnconnected=off
  validOut : Outport  Port=3  VectorParamsAs1DForOutWhenUnconnected=off
  ready : Outport  Port=4  VectorParamsAs1DForOutWhenUnconnected=off
  wires:
  ValidIn to Ready Logic/1(readyOut) -> ready/1
  "CORDIC Reciprocal Normalized, Folded"/4(ready) -> ValidIn to Ready Logic/1(readyIn)
  "CORDIC Reciprocal Normalized, Folded"/2(shift_value) -> shift_value/1
  "CORDIC Reciprocal Normalized, Folded"/3(validOut) -> validOut/1
  validIn/1 -> "CORDIC Reciprocal Normalized, Folded"/2(validIn), ValidIn to Ready Logic/2(validIn)
  x/1 -> y = x(n)/1(x)
  "CORDIC Reciprocal Normalized, Folded"/1(1/x_normalized) -> 1/x_normalized/1
  y = x(n)/1(y) -> "CORDIC Reciprocal Normalized, Folded"/1(x)

== system TxSteering_RxMVDR_4x4_HDL_IQ/DUT/MVDR/Compute Weight Vector/Matrix Left Divide/CORDIC/4x4 Complex CORDIC Matrix Left Divide/Back Substitute 4x4 Complex CORDIC/Invert first element - Folded2 ==
  x : Inport
  validIn : Inport  Port=2
  "CORDIC Reciprocal Normalized, Folded" : Subsystem  TreatAsAtomicUnit=on  mask{NumberOfCORDICIterations=NumberOfCORDICIterations}
      mask prompts: NumberOfCORDICIterations "Number of CORDIC Iterations"
  State Control : StateControl  StateControl=Synchronous
  ValidIn to Ready Logic : Subsystem
  y = x(n) : MATLAB Function  TreatAsAtomicUnit=on  mask{n=1}
  1/x_normalized : Outport  VectorParamsAs1DForOutWhenUnconnected=off
  shift_value : Outport  Port=2  VectorParamsAs1DForOutWhenUnconnected=off
  validOut : Outport  Port=3  VectorParamsAs1DForOutWhenUnconnected=off
  ready : Outport  Port=4  VectorParamsAs1DForOutWhenUnconnected=off
  wires:
  y = x(n)/1(y) -> "CORDIC Reciprocal Normalized, Folded"/1(x)
  "CORDIC Reciprocal Normalized, Folded"/1(1/x_normalized) -> 1/x_normalized/1
  x/1 -> y = x(n)/1(x)
  validIn/1 -> ValidIn to Ready Logic/2(validIn), "CORDIC Reciprocal Normalized, Folded"/2(validIn)
  "CORDIC Reciprocal Normalized, Folded"/3(validOut) -> validOut/1
  "CORDIC Reciprocal Normalized, Folded"/2(shift_value) -> shift_value/1
  "CORDIC Reciprocal Normalized, Folded"/4(ready) -> ValidIn to Ready Logic/1(readyIn)
  ValidIn to Ready Logic/1(readyOut) -> ready/1

== system TxSteering_RxMVDR_4x4_HDL_IQ/DUT/MVDR/Compute Weight Vector/Matrix Left Divide/CORDIC/4x4 Complex CORDIC Matrix Left Divide/Back Substitute 4x4 Complex CORDIC/Invert first element - Folded3 ==
  x : Inport
  validIn : Inport  Port=2
  "CORDIC Reciprocal Normalized, Folded" : Subsystem  TreatAsAtomicUnit=on  mask{NumberOfCORDICIterations=NumberOfCORDICIterations}
      mask prompts: NumberOfCORDICIterations "Number of CORDIC Iterations"
  State Control : StateControl  StateControl=Synchronous
  ValidIn to Ready Logic : Subsystem
  y = x(n) : MATLAB Function  TreatAsAtomicUnit=on  mask{n=1}
  1/x_normalized : Outport  VectorParamsAs1DForOutWhenUnconnected=off
  shift_value : Outport  Port=2  VectorParamsAs1DForOutWhenUnconnected=off
  validOut : Outport  Port=3  VectorParamsAs1DForOutWhenUnconnected=off
  ready : Outport  Port=4  VectorParamsAs1DForOutWhenUnconnected=off
  wires:
  y = x(n)/1(y) -> "CORDIC Reciprocal Normalized, Folded"/1(x)
  "CORDIC Reciprocal Normalized, Folded"/1(1/x_normalized) -> 1/x_normalized/1
  x/1 -> y = x(n)/1(x)
  validIn/1 -> ValidIn to Ready Logic/2(validIn), "CORDIC Reciprocal Normalized, Folded"/2(validIn)
  "CORDIC Reciprocal Normalized, Folded"/3(validOut) -> validOut/1
  "CORDIC Reciprocal Normalized, Folded"/2(shift_value) -> shift_value/1
  "CORDIC Reciprocal Normalized, Folded"/4(ready) -> ValidIn to Ready Logic/1(readyIn)
  ValidIn to Ready Logic/1(readyOut) -> ready/1

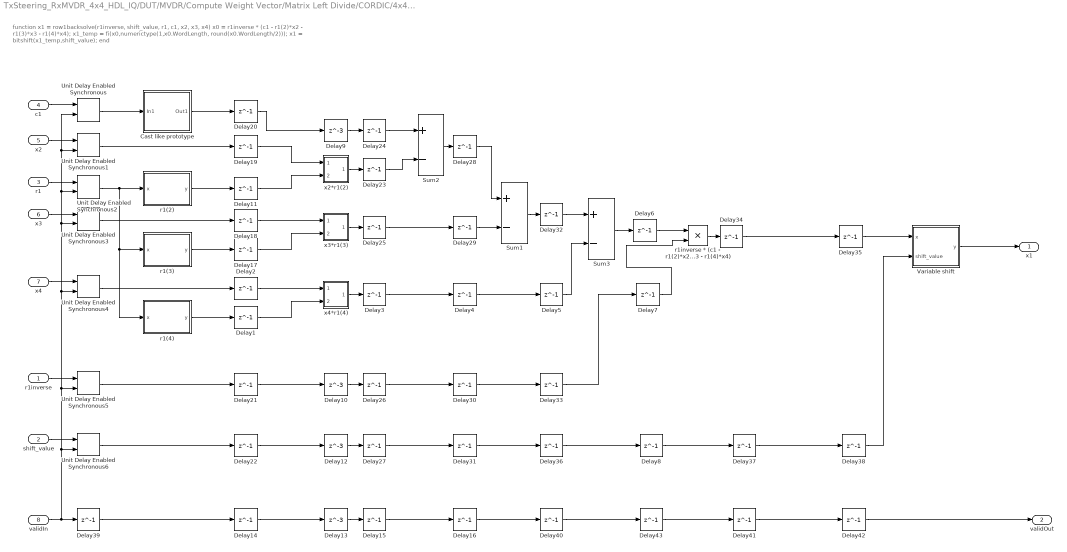
== system TxSteering_RxMVDR_4x4_HDL_IQ/DUT/MVDR/Compute Weight Vector/Matrix Left Divide/CORDIC/4x4 Complex CORDIC Matrix Left Divide/Back Substitute 4x4 Complex CORDIC/Row1 Back Substitute Specify Output Type ==
  note: function x1 = row1backsolve(r1inverse, shift_value, r1, c1, x2, x3, x4)
      | x0 = r1inverse * (c1 - r1(2)*x2 - r1(3)*x3 - r1(4)*x4);
      | x1_temp = fi(x0,numerictype(1,x0.WordLength, round(x0.WordLength/2)));
      | x1 = bitshift(x1_temp,shift_value);
      | end
  r1inverse : Inport
  shift_value : Inport  Port=2
  r1 : Inport  Port=3
  c1 : Inport  Port=4
  x2 : Inport  Port=5
  x3 : Inport  Port=6
  x4 : Inport  Port=7
  validIn : Inport  Port=8
  Cast like prototype : Subsystem  TreatAsAtomicUnit=on  mask{OutputPrototype=OutputPrototype}
      mask prompts: OutputPrototype "Output prototype"
  Delay{1..8,11,14..43} (39 alike) : Delay  DelayLength=1
  Delay{9..10,12..13} (4 alike) : Delay  DelayLength=3
  Sum1 : Sum  Inputs=+-
  Sum2 : Sum  Inputs=+-
  Sum3 : Sum  Inputs=+-
  Unit Delay Enabled Synchronous{,1..6} (7 alike) : hdlsllib/Discrete/Unit Delay Enabled Synchronous  InitialCondition=0.0  SampleTime=-1
      settings: SourceProductBaseCode=SL
  Variable shift : Subsystem  TreatAsAtomicUnit=on
  r1(2) : MATLAB Function  TreatAsAtomicUnit=on  mask{n=2}
  r1(3) : MATLAB Function  TreatAsAtomicUnit=on  mask{n=3}
  r1(4) : MATLAB Function  TreatAsAtomicUnit=on  mask{n=4}
  r1inverse * (c1 - r1(2)*x2 - r1(3)*x3 - r1(4)*x4) : Product  OutDataTypeStr=Inherit: Same as first input
  x2*r1(2) : Subsystem  TreatAsAtomicUnit=on
  x3*r1(3) : Subsystem  TreatAsAtomicUnit=on
  x4*r1(4) : Subsystem  TreatAsAtomicUnit=on
  x1 : Outport  VectorParamsAs1DForOutWhenUnconnected=off
  validOut : Outport  Port=2  VectorParamsAs1DForOutWhenUnconnected=off
  wires:
  Cast like prototype/1(Out1) -> Delay20/1
  Delay34/1 -> Delay35/1
  Delay39/1 -> Delay14/1
  shift_value/1 -> Unit Delay Enabled Synchronous6/1
  Unit Delay Enabled Synchronous6/1 -> Delay22/1
  r1inverse/1 -> Unit Delay Enabled Synchronous5/1
  Unit Delay Enabled Synchronous5/1 -> Delay21/1
  x4/1 -> Unit Delay Enabled Synchronous4/1
  Unit Delay Enabled Synchronous4/1 -> Delay2/1
  x3/1 -> Unit Delay Enabled Synchronous3/1
  Unit Delay Enabled Synchronous3/1 -> Delay18/1
  r1/1 -> Unit Delay Enabled Synchronous2/1
  Unit Delay Enabled Synchronous2/1 -> r1(2)/1(x), r1(4)/1(x), r1(3)/1(x)
  x2/1 -> Unit Delay Enabled Synchronous1/1
  Unit Delay Enabled Synchronous1/1 -> Delay19/1
  c1/1 -> Unit Delay Enabled Synchronous/1
  Unit Delay Enabled Synchronous/1 -> Cast like prototype/1(In1)
  Delay42/1 -> validOut/1
  Delay14/1 -> Delay13/1
  Delay15/1 -> Delay16/1
  Delay41/1 -> Delay42/1
  Delay16/1 -> Delay40/1
  validIn/1 -> Delay39/1, Unit Delay Enabled Synchronous/2, Unit Delay Enabled Synchronous1/2, Unit Delay Enabled Synchronous2/2, Unit Delay Enabled Synchronous3/2, Unit Delay Enabled Synchronous4/2, Unit Delay Enabled Synchronous5/2, Unit Delay Enabled Synchronous6/2
  Delay13/1 -> Delay15/1
  Delay43/1 -> Delay41/1
  Delay40/1 -> Delay43/1
  Variable shift/1(y) -> x1/1
  Delay22/1 -> Delay12/1
  Sum2/1 -> Delay28/1
  x3*r1(3)/1(Out1) -> Delay25/1
  Delay23/1 -> Sum2/2
  Delay38/1 -> Variable shift/2(shift_value)
  r1(3)/1(y) -> Delay17/1
  x2*r1(2)/1(Out1) -> Delay23/1
  Delay11/1 -> x2*r1(2)/2(In2)
  Delay18/1 -> x3*r1(3)/1(In1)
  r1inverse * (c1 - r1(2)*x2 - r1(3)*x3 - r1(4)*x4)/1 -> Delay34/1
  Delay26/1 -> Delay30/1
  Delay20/1 -> Delay9/1
  r1(2)/1(y) -> Delay11/1
  Delay25/1 -> Delay29/1
  Delay24/1 -> Sum2/1
  Delay27/1 -> Delay31/1
  Delay19/1 -> x2*r1(2)/1(In1)
  Sum1/1 -> Delay32/1
  Delay28/1 -> Sum1/1
  Delay30/1 -> Delay33/1
  Delay37/1 -> Delay38/1
  Delay29/1 -> Sum1/2
  Delay21/1 -> Delay10/1
  Delay31/1 -> Delay36/1
  Delay35/1 -> Variable shift/1(x)
  Delay36/1 -> Delay8/1
  Delay17/1 -> x3*r1(3)/2(In2)
  x4*r1(4)/1(Out1) -> Delay3/1
  Delay1/1 -> x4*r1(4)/2(In2)
  r1(4)/1(y) -> Delay1/1
  Delay2/1 -> x4*r1(4)/1(In1)
  Delay3/1 -> Delay4/1
  Delay32/1 -> Sum3/1
  Delay4/1 -> Delay5/1
  Sum3/1 -> Delay6/1
  Delay5/1 -> Sum3/2
  Delay33/1 -> Delay7/1
  Delay6/1 -> r1inverse * (c1 - r1(2)*x2 - r1(3)*x3 - r1(4)*x4)/1
  Delay7/1 -> r1inverse * (c1 - r1(2)*x2 - r1(3)*x3 - r1(4)*x4)/2
  Delay9/1 -> Delay24/1
  Delay10/1 -> Delay26/1
  Delay12/1 -> Delay27/1
  Delay8/1 -> Delay37/1

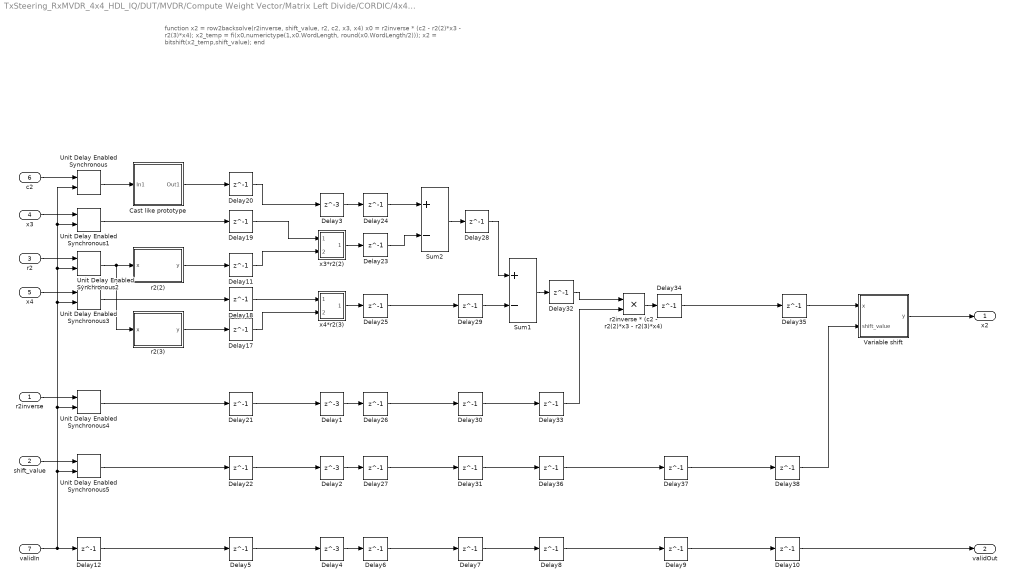
== system TxSteering_RxMVDR_4x4_HDL_IQ/DUT/MVDR/Compute Weight Vector/Matrix Left Divide/CORDIC/4x4 Complex CORDIC Matrix Left Divide/Back Substitute 4x4 Complex CORDIC/Row2 Back Substitute Specify Output Type ==
  note: function x2 = row2backsolve(r2inverse, shift_value, r2, c2, x3, x4)
      | x0 = r2inverse * (c2 - r2(2)*x3 - r2(3)*x4);
      | x2_temp = fi(x0,numerictype(1,x0.WordLength, round(x0.WordLength/2)));
      | x2 = bitshift(x2_temp,shift_value);
      | end
  r2inverse : Inport
  shift_value : Inport  Port=2
  r2 : Inport  Port=3
  x3 : Inport  Port=4
  x4 : Inport  Port=5
  c2 : Inport  Port=6
  validIn : Inport  Port=7
  Cast like prototype : Subsystem  TreatAsAtomicUnit=on  mask{OutputPrototype=OutputPrototype}
      mask prompts: OutputPrototype "Output prototype"
  Delay{1..4} (4 alike) : Delay  DelayLength=3
  Delay{5..12,17..38} (30 alike) : Delay  DelayLength=1
  Sum1 : Sum  Inputs=+-
  Sum2 : Sum  Inputs=+-
  Unit Delay Enabled Synchronous{,1..5} (6 alike) : hdlsllib/Discrete/Unit Delay Enabled Synchronous  InitialCondition=0.0  SampleTime=-1
      settings: SourceProductBaseCode=SL
  Variable shift : Subsystem  TreatAsAtomicUnit=on
  r2(2) : MATLAB Function  TreatAsAtomicUnit=on  mask{n=2}
  r2(3) : MATLAB Function  TreatAsAtomicUnit=on  mask{n=3}
  r2inverse * (c2 - r2(2)*x3 - r2(3)*x4) : Product  OutDataTypeStr=Inherit: Same as first input
  x3*r2(2) : Subsystem  TreatAsAtomicUnit=on
  x4*r2(3) : Subsystem  TreatAsAtomicUnit=on
  x2 : Outport  VectorParamsAs1DForOutWhenUnconnected=off
  validOut : Outport  Port=2  VectorParamsAs1DForOutWhenUnconnected=off
  wires:
  Delay34/1 -> Delay35/1
  Cast like prototype/1(Out1) -> Delay20/1
  Delay12/1 -> Delay5/1
  shift_value/1 -> Unit Delay Enabled Synchronous5/1
  r2inverse/1 -> Unit Delay Enabled Synchronous4/1
  Unit Delay Enabled Synchronous5/1 -> Delay22/1
  Unit Delay Enabled Synchronous4/1 -> Delay21/1
  x4/1 -> Unit Delay Enabled Synchronous3/1
  Unit Delay Enabled Synchronous3/1 -> Delay18/1
  r2/1 -> Unit Delay Enabled Synchronous2/1
  Unit Delay Enabled Synchronous2/1 -> r2(2)/1(x), r2(3)/1(x)
  x3/1 -> Unit Delay Enabled Synchronous1/1
  Unit Delay Enabled Synchronous1/1 -> Delay19/1
  c2/1 -> Unit Delay Enabled Synchronous/1
  Unit Delay Enabled Synchronous/1 -> Cast like prototype/1(In1)
  Delay10/1 -> validOut/1
  Delay8/1 -> Delay9/1
  Delay4/1 -> Delay6/1
  Delay9/1 -> Delay10/1
  Delay7/1 -> Delay8/1
  Delay5/1 -> Delay4/1
  Delay6/1 -> Delay7/1
  validIn/1 -> Delay12/1, Unit Delay Enabled Synchronous/2, Unit Delay Enabled Synchronous1/2, Unit Delay Enabled Synchronous2/2, Unit Delay Enabled Synchronous3/2, Unit Delay Enabled Synchronous4/2, Unit Delay Enabled Synchronous5/2
  Delay36/1 -> Delay37/1
  Delay3/1 -> Delay24/1
  Delay2/1 -> Delay27/1
  Delay1/1 -> Delay26/1
  Variable shift/1(y) -> x2/1
  Delay38/1 -> Variable shift/2(shift_value)
  Delay37/1 -> Delay38/1
  Delay35/1 -> Variable shift/1(x)
  Delay33/1 -> r2inverse * (c2 - r2(2)*x3 - r2(3)*x4)/2
  Delay32/1 -> r2inverse * (c2 - r2(2)*x3 - r2(3)*x4)/1
  Delay31/1 -> Delay36/1
  Delay30/1 -> Delay33/1
  Delay29/1 -> Sum1/2
  Delay28/1 -> Sum1/1
  Sum2/1 -> Delay28/1
  Delay27/1 -> Delay31/1
  Delay26/1 -> Delay30/1
  Delay25/1 -> Delay29/1
  Delay24/1 -> Sum2/1
  Delay23/1 -> Sum2/2
  x3*r2(2)/1(Out1) -> Delay23/1
  Delay22/1 -> Delay2/1
  Delay21/1 -> Delay1/1
  Delay20/1 -> Delay3/1
  r2inverse * (c2 - r2(2)*x3 - r2(3)*x4)/1 -> Delay34/1
  Sum1/1 -> Delay32/1
  x4*r2(3)/1(Out1) -> Delay25/1
  Delay17/1 -> x4*r2(3)/2(In2)
  Delay18/1 -> x4*r2(3)/1(In1)
  Delay11/1 -> x3*r2(2)/2(In2)
  Delay19/1 -> x3*r2(2)/1(In1)
  r2(3)/1(y) -> Delay17/1
  r2(2)/1(y) -> Delay11/1

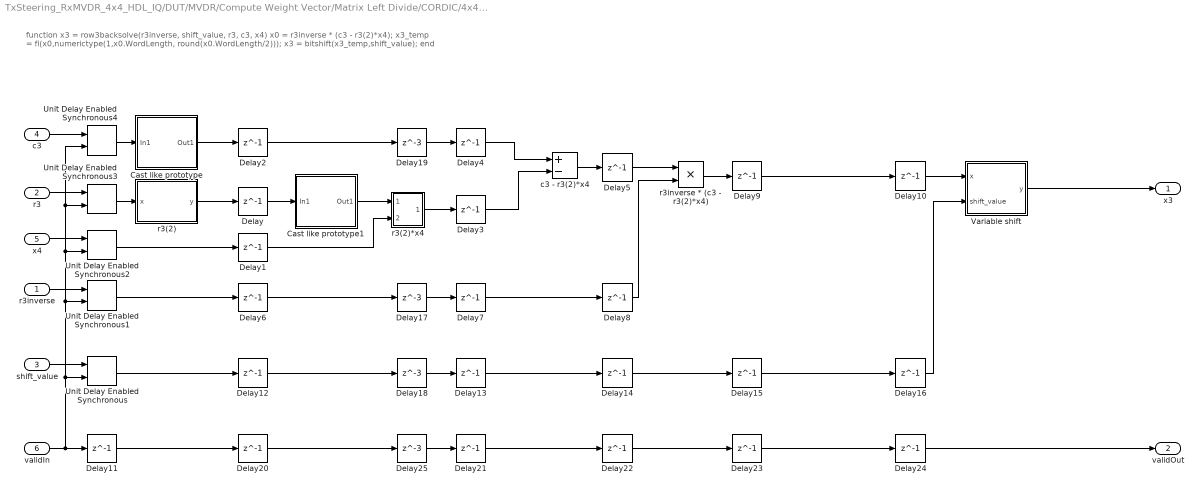
== system TxSteering_RxMVDR_4x4_HDL_IQ/DUT/MVDR/Compute Weight Vector/Matrix Left Divide/CORDIC/4x4 Complex CORDIC Matrix Left Divide/Back Substitute 4x4 Complex CORDIC/Row3 Back Substitute Specify Output Type ==
  note: function x3 = row3backsolve(r3inverse, shift_value, r3, c3, x4)
      | x0 = r3inverse * (c3 - r3(2)*x4);
      | x3_temp = fi(x0,numerictype(1,x0.WordLength, round(x0.WordLength/2)));
      | x3 = bitshift(x3_temp,shift_value);
      | end
  r3inverse : Inport
  r3 : Inport  Port=2
  shift_value : Inport  Port=3
  c3 : Inport  Port=4
  x4 : Inport  Port=5
  validIn : Inport  Port=6
  Cast like prototype : Subsystem  TreatAsAtomicUnit=on  mask{OutputPrototype=OutputPrototype}
      mask prompts: OutputPrototype "Output prototype"
  Cast like prototype1 : Subsystem  TreatAsAtomicUnit=on  mask{OutputPrototype=OutputPrototype}
      mask prompts: OutputPrototype "Output prototype"
  Delay{,1..16,20..24} (22 alike) : Delay  DelayLength=1
  Delay{17..19,25} (4 alike) : Delay  DelayLength=3
  Unit Delay Enabled Synchronous{,1..4} (5 alike) : hdlsllib/Discrete/Unit Delay Enabled Synchronous  InitialCondition=0.0  SampleTime=-1
      settings: SourceProductBaseCode=SL
  Variable shift : Subsystem  TreatAsAtomicUnit=on
  c3 - r3(2)*x4 : Sum  Inputs=+-
  r3(2) : MATLAB Function  TreatAsAtomicUnit=on  mask{n=2}
  r3(2)*x4 : Subsystem  TreatAsAtomicUnit=on
  r3inverse * (c3 - r3(2)*x4) : Product  OutDataTypeStr=Inherit: Same as first input
  x3 : Outport  VectorParamsAs1DForOutWhenUnconnected=off
  validOut : Outport  Port=2  VectorParamsAs1DForOutWhenUnconnected=off
  wires:
  Delay2/1 -> Delay19/1
  Cast like prototype1/1(Out1) -> r3(2)*x4/1(In1)
  Delay9/1 -> Delay10/1
  Cast like prototype/1(Out1) -> Delay2/1
  shift_value/1 -> Unit Delay Enabled Synchronous/1
  r3inverse/1 -> Unit Delay Enabled Synchronous1/1
  x4/1 -> Unit Delay Enabled Synchronous2/1
  r3/1 -> Unit Delay Enabled Synchronous3/1
  c3/1 -> Unit Delay Enabled Synchronous4/1
  Delay11/1 -> Delay20/1
  Unit Delay Enabled Synchronous/1 -> Delay12/1
  Unit Delay Enabled Synchronous1/1 -> Delay6/1
  Unit Delay Enabled Synchronous2/1 -> Delay1/1
  Unit Delay Enabled Synchronous3/1 -> r3(2)/1(x)
  Unit Delay Enabled Synchronous4/1 -> Cast like prototype/1(In1)
  Delay24/1 -> validOut/1
  Delay20/1 -> Delay25/1
  Delay21/1 -> Delay22/1
  Delay25/1 -> Delay21/1
  validIn/1 -> Delay11/1, Unit Delay Enabled Synchronous4/2, Unit Delay Enabled Synchronous3/2, Unit Delay Enabled Synchronous2/2, Unit Delay Enabled Synchronous1/2, Unit Delay Enabled Synchronous/2
  Delay23/1 -> Delay24/1
  Delay22/1 -> Delay23/1
  Delay19/1 -> Delay4/1
  Delay1/1 -> r3(2)*x4/2(In2)
  Delay8/1 -> r3inverse * (c3 - r3(2)*x4)/2
  Delay14/1 -> Delay15/1
  Delay18/1 -> Delay13/1
  Delay17/1 -> Delay7/1
  Delay13/1 -> Delay14/1
  Delay16/1 -> Variable shift/2(shift_value)
  Delay15/1 -> Delay16/1
  Delay12/1 -> Delay18/1
  Variable shift/1(y) -> x3/1
  Delay10/1 -> Variable shift/1(x)
  r3inverse * (c3 - r3(2)*x4)/1 -> Delay9/1
  Delay7/1 -> Delay8/1
  Delay6/1 -> Delay17/1
  Delay5/1 -> r3inverse * (c3 - r3(2)*x4)/1
  c3 - r3(2)*x4/1 -> Delay5/1
  Delay3/1 -> c3 - r3(2)*x4/2
  Delay4/1 -> c3 - r3(2)*x4/1
  r3(2)*x4/1(Out1) -> Delay3/1
  Delay/1 -> Cast like prototype1/1(In1)
  r3(2)/1(y) -> Delay/1

== system TxSteering_RxMVDR_4x4_HDL_IQ/DUT/MVDR/Compute Weight Vector/Matrix Left Divide/CORDIC/4x4 Complex CORDIC Matrix Left Divide/Back Substitute 4x4 Complex CORDIC/Row4 Back Substitute Specify Output Type ==
  note: function x4 = row4backsolve(r4inverse, shift_value, c4)
      | x0 = r4inverse * c4;
      | x4_temp = fi(x0,numerictype(1,x0.WordLength, round(x0.WordLength/2)));
      | x4 = bitshift(x4_temp,shift_value);
      | end
  r4inverse : Inport
  shift_value : Inport  Port=2
  c4 : Inport  Port=3
  validIn : Inport  Port=4
  Cast like prototype : Subsystem  TreatAsAtomicUnit=on  mask{OutputPrototype=OutputPrototype}
      mask prompts: OutputPrototype "Output prototype"
  Delay : Delay  DelayLength=1
  Delay1 : Delay  DelayLength=1
  Delay2 : Delay  DelayLength=1
  Product : Product  OutDataTypeStr=Inherit: Same as first input
  Unit Delay Enabled Synchronous : hdlsllib/Discrete/Unit Delay Enabled Synchronous  InitialCondition=0.0  SampleTime=-1
      settings: SourceProductBaseCode=SL
  Unit Delay Enabled Synchronous1 : hdlsllib/Discrete/Unit Delay Enabled Synchronous  InitialCondition=0.0  SampleTime=-1
      settings: SourceProductBaseCode=SL
  Unit Delay Enabled Synchronous2 : hdlsllib/Discrete/Unit Delay Enabled Synchronous  InitialCondition=0.0  SampleTime=-1
      settings: SourceProductBaseCode=SL
  Variable shift : Subsystem  TreatAsAtomicUnit=on
  x4 : Outport  VectorParamsAs1DForOutWhenUnconnected=off
  validOut : Outport  Port=2  VectorParamsAs1DForOutWhenUnconnected=off
  wires:
  Delay1/1 -> Delay2/1
  validIn/1 -> Delay1/1, Unit Delay Enabled Synchronous2/2, Unit Delay Enabled Synchronous1/2, Unit Delay Enabled Synchronous/2
  c4/1 -> Unit Delay Enabled Synchronous2/1
  Unit Delay Enabled Synchronous2/1 -> Product/1
  Unit Delay Enabled Synchronous1/1 -> Product/2
  r4inverse/1 -> Unit Delay Enabled Synchronous1/1
  Unit Delay Enabled Synchronous/1 -> Variable shift/2(shift_value)
  shift_value/1 -> Unit Delay Enabled Synchronous/1
  Delay2/1 -> validOut/1
  Variable shift/1(y) -> x4/1
  Delay/1 -> Variable shift/1(x)
  Cast like prototype/1(Out1) -> Delay/1
  Product/1 -> Cast like prototype/1(In1)
